simulink library "lib_Convection_FluidEnergyBalance"  (R2015a)
settings: Solver=ode45  StartTime=0.0  StopTime=10.0  RelTol=1e-3
libraries: simulink x1
settings Model: Creator=jlkratz  LastModifiedBy=jlkratz

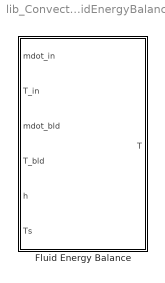
== system lib_Convection_FluidEnergyBalance ==
  Fluid Energy Balance : Subsystem  mask(TSAT: Fluid Energy Balance){x_M=linspace(0,5,500), As_M=0.05*ones(1,500), Blds_M=on, xbld_M=[2 4], CpData_M=[5998.8 6008.2 6152.8 6443.4 6736.5 6972.4 7151.4 7288.1 7395.4 7482.5], TData_M=[100 497.8 885.56 1273.3 1661.1 2048.9 2436.7 2824.4 3212.2 3600], Tin0_M=550, BN_M=double(gcb)}
      mask prompts: x_M "x_M - Array of discretized x-locations [Nx1]"; As_M "As_M - Array of discretized surface areas participating in heat transfer [NxM]"; Blds_M "Blds_M - Checked if there are bleeds, unchecked otherwise"; xbld_M "xbld_M - Location of bleeds in the x-domain [nx1]"; CpData_M "CpData_M - Heat capacity array for interpolation [mx1]"; TData_M "TData_M - Temperature array for interpolation of the heat capacity [mx1]"; Tin0_M "Tin0_M - Initial inlet temperature (used to initialize Cp) [1x1]"; BN_M "BN_M - Block name"
      mask help:
      | This block attempts to approximate the steady-state temperature of a fluid flowing through a path that is heated/cooled by the solid surfaces that enclose the fluid. The approximation is made by breaking the domain in the flow direction up into a number of control volumes. Then a simple energy balance is performed for each volume starting with the most upstream and ending with the most downstream. The energy equation comes straight from basic thermodynamics. This block neglects potential energy due to gravity, local kinetic energy as a result of the fluids velocity, and the addition of work. This leaves the main contributors to be enthalpy of the fluid and heat transfer from adjacent surfaces. This makes this block most appropriate for flows which the effects of gravity is negligible, the flow is moving at a relatively low speed there is no work addition/extraction, but there is significant heat transfer.
      |
      | See the block help menu for more details.
      mask init:
      | %setup inports ===========================================================%
      | 
      | % Inport Numbers
      | n = 3;
      | 
      | %mdot_bld
      | % Bleed mass flow rate(s)
      | if Blds_M == 1
      |     if strcmp(get_param([BN_M '/mdot_bld'],'BlockType'),'Constant')
      |         MSK_ReplaceBlock_TSAT([BN_M '/mdot_bld'],'built-in/Inport');
      |     end
      |     set_param([BN_M '/mdot_bld'],'Port',num2str(n));
      |     n = n + 1;
      | elseif Blds_M == 0
      |     if strcmp(get_param([BN_M '/mdot_bld'],'BlockType'),'Inport')
      |         MSK_ReplaceBlock_TSAT([BN_M '/mdot_bld'],'built-in/Constant');
      |         set_param([BN_M '/mdot_bld'],'Value','0');
      |     end
      | end
      | 
      | %mdot_bld
      | % Bleed Temperature(s)
      | if Blds_M == 1
      |     if strcmp(get_param([BN_M '/T_bld'],'BlockType'),'Constant')
      |         MSK_ReplaceBlock_TSAT([BN_M '/T_bld'],'built-in/Inport');
      |     end
      |     set_param([BN_M '/T_bld'],'Port',num2str(n));
      |     n = n + 1;
      | elseif Blds_M == 0
      |     if strcmp(get_param([BN_M '/T_bld'],'BlockType'),'Inport')
      |         MSK_ReplaceBlock_TSAT([BN_M '/T_bld'],'built-in/Constant');
      |         set_param([BN_M '/T_bld'],'Value','0');
      |     end
      | end
      | 
      | if Blds_M == 0
      |     xbld_M = 0;
      | end
      mask Help: web(which('Convection_TSAT_FluidEnergyBalance.html'),'-helpbrowser')
      mask Callback Blds_M:
      | opt = get_param(gcb,'Blds_M');
      | if opt(2) == 'n' %on vs. off
      |     MSK_SEC_Enables2_TSAT('Blds_M',4,'en');
      | else
      |     MSK_SEC_Enables2_TSAT('Blds_M',4,'dis');
      | end
      | clear opt
      mask DialogControl Container3 Prompt: Discretization arrays
      mask DialogControl Container4 Prompt: Bleeds
      mask DialogControl Container5 Prompt: Gas Properties

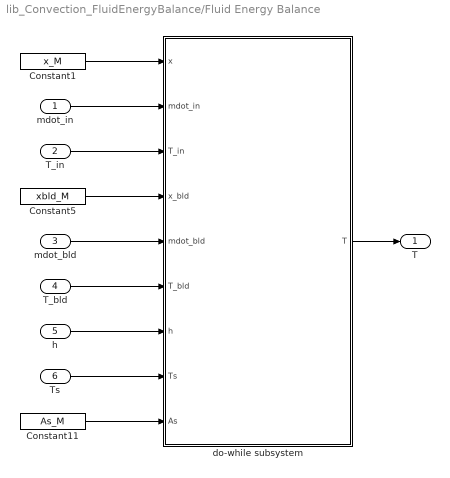
== system lib_Convection_FluidEnergyBalance/Fluid Energy Balance ==
  mdot_in : Inport
  T_in : Inport  Port=2
  mdot_bld : Inport  Port=3
  T_bld : Inport  Port=4
  h : Inport  Port=5
  Ts : Inport  Port=6
  Constant1 : Constant  Value=x_M
  Constant11 : Constant  Value=As_M
  Constant5 : Constant  Value=xbld_M
  do-while subsystem : Subsystem
  T : Outport
  wires:
  do-while subsystem/1(T) -> T/1
  Constant11/1 -> do-while subsystem/9(As)
  Ts/1 -> do-while subsystem/8(Ts)
  h/1 -> do-while subsystem/7(h)
  T_bld/1 -> do-while subsystem/6(T_bld)
  mdot_bld/1 -> do-while subsystem/5(mdot_bld)
  Constant5/1 -> do-while subsystem/4(x_bld)
  T_in/1 -> do-while subsystem/3(T_in)
  mdot_in/1 -> do-while subsystem/2(mdot_in)
  Constant1/1 -> do-while subsystem/1(x)

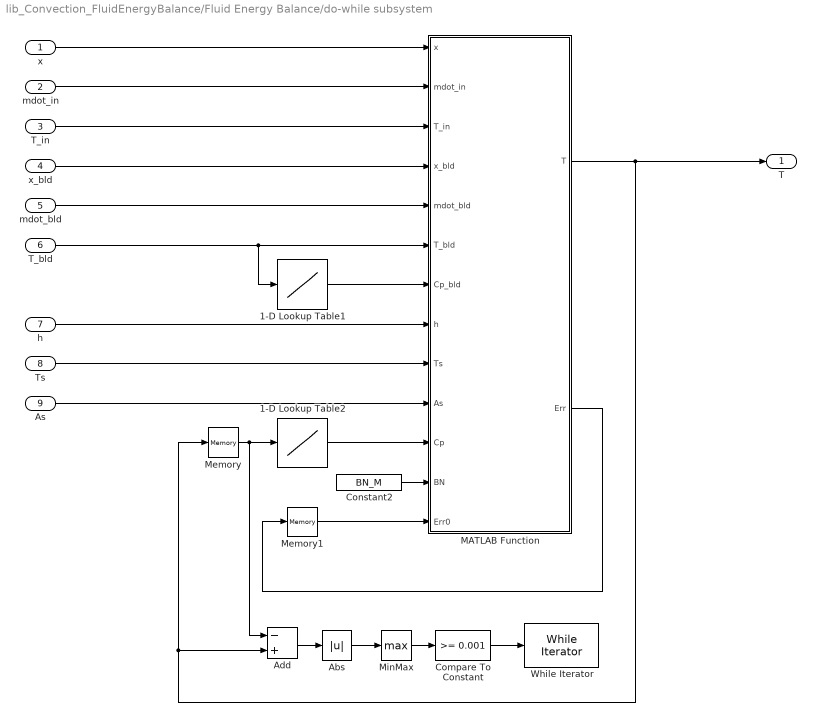
== system lib_Convection_FluidEnergyBalance/Fluid Energy Balance/do-while subsystem ==
  x : Inport
  mdot_in : Inport  Port=2
  T_in : Inport  Port=3
  x_bld : Inport  Port=4
  mdot_bld : Inport  Port=5
  T_bld : Inport  Port=6
  h : Inport  Port=7
  Ts : Inport  Port=8
  As : Inport  Port=9
  1-D Lookup Table1 : Lookup_n-D  NumberOfTableDimensions=1  BreakpointsForDimension1=TData_M  Table=CpData_M  InternalRulePriority=Speed  RndMeth=Simplest  InputSameDT=on
  1-D Lookup Table2 : Lookup_n-D  NumberOfTableDimensions=1  BreakpointsForDimension1=TData_M  Table=CpData_M  InternalRulePriority=Speed  RndMeth=Simplest  InputSameDT=on
  Abs : Abs
  Add : Sum  Inputs=-+
  Compare To Constant : simulink/Logic and Bit Operations/Compare To Constant  relop=>=  const=0.001  OutDataTypeStr=boolean
  Constant2 : Constant  Value=BN_M
  MATLAB Function : MATLAB Function  TreatAsAtomicUnit=on
  Memory : Memory  X0=Tin0_M*ones(1,length(x_M))  InheritSampleTime=on
  Memory1 : Memory  X0=zeros(1,37)  InheritSampleTime=on
  MinMax : MinMax  Function=max
  While Iterator : WhileIterator  MaxIters=1000  WhileBlockType=do-while
  T : Outport
  wires:
  MinMax/1 -> Compare To Constant/1
  Add/1 -> Abs/1
  Compare To Constant/1 -> While Iterator/1
  Abs/1 -> MinMax/1
  MATLAB Function/2(Err) -> Memory1/1
  Memory1/1 -> MATLAB Function/13(Err0)
  1-D Lookup Table2/1 -> MATLAB Function/11(Cp)
  1-D Lookup Table1/1 -> MATLAB Function/7(Cp_bld)
  As/1 -> MATLAB Function/10(As)
  Memory/1 -> 1-D Lookup Table2/1, Add/1
  Ts/1 -> MATLAB Function/9(Ts)
  MATLAB Function/1(T) -> Memory/1, Add/2, T/1
  h/1 -> MATLAB Function/8(h)
  x_bld/1 -> MATLAB Function/4(x_bld)
  T_bld/1 -> MATLAB Function/6(T_bld), 1-D Lookup Table1/1
  T_in/1 -> MATLAB Function/3(T_in)
  mdot_in/1 -> MATLAB Function/2(mdot_in)
  mdot_bld/1 -> MATLAB Function/5(mdot_bld)
  x/1 -> MATLAB Function/1(x)
  Constant2/1 -> MATLAB Function/12(BN)

== matlab function lib_Convection_FluidEnergyBalance/Fluid Energy Balance/do-while subsystem/MATLAB Function ==
  data: x input; T output; mdot_in input; T_in input; x_bld input; mdot_bld input; T_bld input; Cp_bld input; h input; Ts input; As input; Cp input; BN input; Err0 input; Err output
function [T,Err] = FlowEnergyBal(x,mdot_in,T_in,x_bld,mdot_bld,T_bld,Cp_bld,h,Ts,As,Cp,BN,Err0)
%#codegen

%error/warning checks ----------------------------------------------------%

Err = Err0;
ErrNum = 1;

%---- x ----%
%length > 1?
if length(x) < 2 && Err(ErrNum) < 1
    Err(ErrNum) = 1;
    fprintf('Warning in %s: x_M must be a 1-D array of at least 2 elements.\n',char(BN));
end
ErrNum = ErrNum + 1;
%real?
if min(isreal(x)) < 1 && Err(ErrNum) < 1
    Err(ErrNum) = 1;
    fprintf('Warning in %s: x_M must have all real elements.\n',char(BN));
end
ErrNum = ErrNum + 1;
%finite?
if min(isfinite(x)) < 1 && Err(ErrNum) < 1
    Err(ErrNum) = 1;
    fprintf('Warning in %s: x_M must have all finite elements.\n',char(BN));
end
ErrNum = ErrNum + 1;
%monotonically increasing?
if min(diff(x)) <= 0 && Err(ErrNum) < 1
    Err(ErrNum) = 1;
    fprintf('Warning in %s: x_M must be monotonically increasing.\n',char(BN));
end
ErrNum = ErrNum + 1;

%---- mdot_in ----%
%scalar?
if isscalar(mdot_in) < 1 && Err(ErrNum) < 1
    Err(ErrNum) = 1;
    fprintf('Warning in %s: mdot_in must be a scalar.\n',char(BN));
end
ErrNum = ErrNum + 1;
%real?
if isreal(mdot_in) < 1 && Err(ErrNum) < 1
    Err(ErrNum) = 1;
    fprintf('Warning in %s: mdot_in must be real.\n',char(BN));
end
ErrNum = ErrNum + 1;
%finite?
if isfinite(mdot_in) < 1 && Err(ErrNum) < 1
    Err(ErrNum) = 1;
    fprintf('Warning in %s: mdot_in must be finite.\n',char(BN));
end
ErrNum = ErrNum + 1;
%positive?
if mdot_in <= 0 && Err(ErrNum) < 1
    Err(ErrNum) = 1;
    fprintf('Warning in %s: mdot_in is negative. The inlet mass flow rate must be positive.\n',char(BN));
end
ErrNum = ErrNum + 1;

%---- T_in ----%
%scalar?
if isscalar(T_in) < 1 && Err(ErrNum) < 1
    Err(ErrNum) = 1;
    fprintf('Warning in %s: T_in must be a scalar.\n',char(BN));
end
ErrNum = ErrNum + 1;
%real?
if isreal(T_in) < 1 && Err(ErrNum) < 1
    Err(ErrNum) = 1;
    fprintf('Warning in %s: T_in must be real.\n',char(BN));
end
ErrNum = ErrNum + 1;
%finite?
if isfinite(T_in) < 1 && Err(ErrNum) < 1
    Err(ErrNum) = 1;
    fprintf('Warning in %s: T_in must be finite.\n',char(BN));
end
ErrNum = ErrNum + 1;

%---- x_bld ----%
%real?
if min(isreal(x_bld)) < 1 && Err(ErrNum) < 1
    Err(ErrNum) = 1;
    fprintf('Warning in %s: x_bld must have all real elements.\n',char(BN));
end
ErrNum = ErrNum + 1;
%finite?
if min(isfinite(x_bld)) < 1 && Err(ErrNum) < 1
    Err(ErrNum) = 1;
    fprintf('Warning in %s: x_bld must have all finite elements.\n',char(BN));
end
ErrNum = ErrNum + 1;
%monotonically increasing?
if length(x_bld) > 1
    if min(diff(x_bld)) <= 0 && Err(ErrNum) < 1
        Err(ErrNum) = 1;
        fprintf('Warning in %s: x_bld must be monotonically increasing.\n',char(BN));
    end
end
ErrNum = ErrNum + 1;

%---- mdot_bld ----%
%length of x_bld?
if length(mdot_bld) ~= length(x_bld) && Err(ErrNum) < 1
    Err(ErrNum) = 1;
    fprintf('Warning in %s: mdot_bld must be the same length as x_bld.\n',char(BN));
end
ErrNum = ErrNum + 1;
%real?
if min(isreal(mdot_bld)) < 1 && Err(ErrNum) < 1
    Err(ErrNum) = 1;
    fprintf('Warning in %s: mdot_bld must have all real elements.\n',char(BN));
end
ErrNum = ErrNum + 1;
%finite?
if min(isfinite(mdot_bld)) < 1 && Err(ErrNum) < 1
    Err(ErrNum) = 1;
    fprintf('Warning in %s: mdot_bld must have all finite elements.\n',char(BN));
end
ErrNum = ErrNum + 1;
%---- total mass flow rate must be postive ----%
mdotSUM = zeros(1,length(x_bld));
for i = 1:length(x_bld)
    mdotSUM(i) = mdot_in + sum(mdot_bld(1:i));
end
if min(mdotSUM) <= 0 && Err(ErrNum) < 1
    Err(ErrNum) = 1;
    fprintf('Warning in %s: More fluid is being bled than exists in the flow. One or more of the values of mdot_bld are too negative.\n',char(BN));
end
ErrNum = ErrNum + 1;

%---- T_bld ----%
%length of x_bld?
if length(mdot_bld) ~= length(x_bld) && Err(ErrNum) < 1
    Err(ErrNum) = 1;
    fprintf('Warning in %s: mdot_bld must be the same length as x_bld.\n',char(BN));
end
ErrNum = ErrNum + 1;
%real?
if min(isreal(mdot_bld)) < 1 && Err(ErrNum) < 1
    Err(ErrNum) = 1;
    fprintf('Warning in %s: mdot_bld must have all real elements.\n',char(BN));
end
ErrNum = ErrNum + 1;
%finite?
if min(isfinite(mdot_bld)) < 1 && Err(ErrNum) < 1
    Err(ErrNum) = 1;
    fprintf('Warning in %s: mdot_bld must have all finite elements.\n',char(BN));
end
ErrNum = ErrNum + 1;

%---- Cp_bld ----%
%real?
if min(isreal(Cp_bld)) < 1 && Err(ErrNum) < 1
    Err(ErrNum) = 1;
    fprintf('Warning in %s: Cp_bld must have all real elements. Check values for TData_M, CpData_M, and T_bld.\n',char(BN));
end
ErrNum = ErrNum + 1;
%finite?
if min(isfinite(Cp_bld)) < 1 && Err(ErrNum) < 1
    Err(ErrNum) = 1;
    fprintf('Warning in %s: Cp_bld must have all finite elements.  Check values for TData_M, CpData_M, and T_bld.\n',char(BN));
end
ErrNum = ErrNum + 1;
%positive?
if min(Cp_bld) <= 0 && Err(ErrNum) < 1
    Err(ErrNum) = 1;
    fprintf('Warning in %s: Cp_bld must be postive. Check values for TData_M, CpData_M, and T_bld.\n',char(BN));
end
ErrNum = ErrNum + 1;

%---- As ----%
%# rows = length of x
if size(As,1) ~= length(x) && Err(ErrNum) < 1
    Err(ErrNum) = 1;
    fprintf('Warning in %s: As_M must have as many rows as there are elements in x_M.\n',char(BN));
end
ErrNum = ErrNum + 1;
%real?
if min(min(isreal(As))) < 1 && Err(ErrNum) < 1
    Err(ErrNum) = 1;
    fprintf('Warning in %s: As_M must have all real elements.\n',char(BN));
end
ErrNum = ErrNum + 1;
%finite?
if min(min(isfinite(As))) < 1 && Err(ErrNum) < 1
    Err(ErrNum) = 1;
    fprintf('Warning in %s: As_M must have all finite elements. \n',char(BN));
end
ErrNum = ErrNum + 1;
%positive?
if min(min(As)) <= 0 && Err(ErrNum) < 1
    Err(ErrNum) = 1;
    fprintf('Warning in %s: As_M must have all postive elements.\n',char(BN));
end
ErrNum = ErrNum + 1;

%---- h ----%
%size of As?
if size(h,1) ~= size(As,1) && size(h,2) ~= size(As,2) && Err(ErrNum) < 1
    Err(ErrNum) = 1;
    fprintf('Warning in %s: h must be the same size as As_M.\n',char(BN));
end
ErrNum = ErrNum + 1;
%real?
if min(min(isreal(h))) < 1 && Err(ErrNum) < 1
    Err(ErrNum) = 1;
    fprintf('Warning in %s: h must have all real elements.\n',char(BN));
end
ErrNum = ErrNum + 1;
%finite?
if min(min(isfinite(h))) < 1 && Err(ErrNum) < 1
    Err(ErrNum) = 1;
    fprintf('Warning in %s: h must have all finite elements. \n',char(BN));
end
ErrNum = ErrNum + 1;

%---- Ts ----%
%size of As?
if size(Ts,1) ~= size(As,1) && size(Ts,2) ~= size(As,2) && Err(ErrNum) < 1
    Err(ErrNum) = 1;
    fprintf('Warning in %s: Ts must be the same size as As_M.\n',char(BN));
end
ErrNum = ErrNum + 1;
%real?
if min(min(isreal(Ts))) < 1 && Err(ErrNum) < 1
    Err(ErrNum) = 1;
    fprintf('Warning in %s: Ts must have all real elements.\n',char(BN));
end
ErrNum = ErrNum + 1;
%finite?
if min(min(isfinite(Ts))) < 1 && Err(ErrNum) < 1
    Err(ErrNum) = 1;
    fprintf('Warning in %s: Ts must have all finite elements.\n',char(BN));
end
ErrNum = ErrNum + 1;

%---- Cp ----%
%real?
if min(isreal(Cp)) < 1 && Err(ErrNum) < 1
    Err(ErrNum) = 1;
    fprintf('Warning in %s: Cp must have all real elements. Check values for TData_M, CpData_M, T0_M, and T.\n',char(BN));
end
ErrNum = ErrNum + 1;
%finite?
if min(isfinite(Cp)) < 1 && Err(ErrNum) < 1
    Err(ErrNum) = 1;
    fprintf('Warning in %s: Cp must have all finite elements.  Check values for TData_M, CpData_M, T0_M, and T.\n',char(BN));
end
ErrNum = ErrNum + 1;
%positive?
if min(Cp) <= 0 && Err(ErrNum) < 1
    Err(ErrNum) = 1;
    fprintf('Warning in %s: Cp must be postive. Check values for TData_M, CpData_M, T0_M, and T.\n',char(BN));
end

%calculations ------------------------------------------------------------%

%initialize arrays
mdot = zeros(1,length(x));
T = zeros(1,length(x));
%set first point
mdot(1) = mdot_in;
T(1) = T_in;

%heat transfer components
hAT = zeros(1,length(x));
hA = zeros(1,length(x));
for i = 1:size(h,1)
    hAT(i) = sum(h(i,:).*As(i,:).*Ts(i,:),2);
    hA(i) = sum(h(i,:).*As(i,:),2);
end

%set bleed index
i_bld = 1;
for i = 2:length(x)
    if i_bld <= length(x_bld)
        if x(i) >= x_bld(i_bld)
            mdot(i) = mdot(i-1) + mdot_bld(i_bld);
            if mdot_bld(i_bld) >=0 
                NUM = mdot(i-1)*Cp(i-1)*T(i-1) + mdot_bld(i_bld)*Cp_bld(i_bld)*T_bld(i_bld) + hAT(i);
                DEN = mdot(i-1)*Cp(i) + mdot_bld(i_bld)*Cp(i) + hA(i);
            else
                NUM = mdot(i)*Cp(i-1)*T(i-1) + hAT(i);
                DEN = mdot(i)*Cp(i) + hA(i);
            end
            i_bld = i_bld + 1;
        else
            mdot(i) = mdot(i-1);
            NUM = mdot(i-1)*Cp(i-1)*T(i-1) + hAT(i);
            DEN = mdot(i-1)*Cp(i) + hA(i);
        end
    else
        mdot(i) = mdot(i-1);
        NUM = mdot(i-1)*Cp(i-1)*T(i-1) + hAT(i);
        DEN = mdot(i-1)*Cp(i) + hA(i);
    end
    T(i) = NUM/DEN;
end
